simulink model "anti_condensation_control"  (R2025a)
settings: Solver=FixedStepDiscrete  StartTime=0.0  StopTime=5400  FixedStep=0.5  RelTol=1e-3
model workspace (MAT data in the model file):
  C_th = 700
  P_loss0 = 55
  R_th0 = 0.48
  T_mod0 = 27
  V_max = 880
  V_min = 580
  V_nom = 620
  dT_2nd = 8
  dT_th = 5
  dV_step = 15
  fan_nom = 100
undefined symbols (not defined in the file or in its folder): DiscIntNeverNeededParam
settings Model: Creator=jicai  LastModifiedBy=jicai

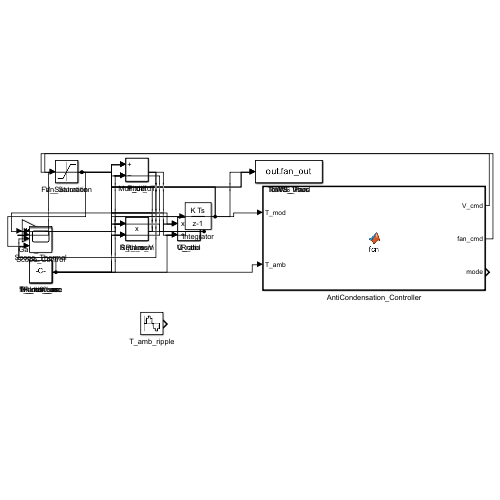
[thumbnail: Simulink's stored preview of the top-level diagram]
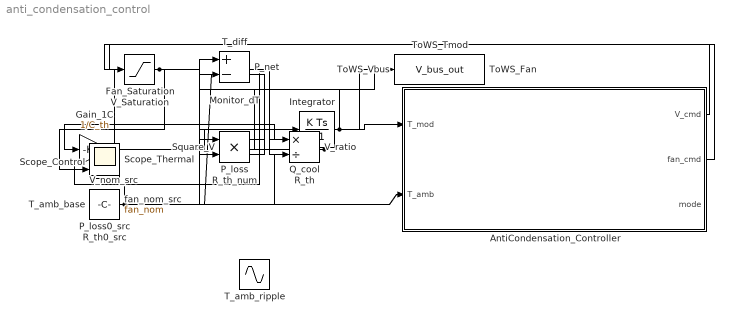
== system anti_condensation_control ==
  AntiCondensation_Controller : MATLAB Function  TreatAsAtomicUnit=on
  Fan_Saturation : Saturate  UpperLimit=100  LowerLimit=15
  Gain_1C : Gain  Gain=1/C_th
  Integrator : DiscreteIntegrator  InitialCondition=T_mod0  SampleTime=0.5  ICPrevOutput=DiscIntNeverNeededParam  ICPrevScaledInput=DiscIntNeverNeededParam
  Monitor_dT : Sum  Inputs=+-
  P_loss : Product  Inputs=**
  P_loss0_src : Constant  Value=P_loss0
  P_net : Sum  Inputs=+-
  Q_cool : Product  Inputs=*/
  R_th : Product  Inputs=*/
  R_th0_src : Constant  Value=R_th0
  R_th_num : Product  Inputs=**
  Scope_Control : Scope  NumInputPorts=2
  Scope_Thermal : Scope  NumInputPorts=3
  Square_V : Product  Inputs=**
  T_amb_base : Constant  Value=38
  T_amb_ripple : Sin  Amplitude=1.2  Frequency=0.00628  SampleTime=0.5
  T_diff : Sum  Inputs=+-
  ToWS_Fan : ToWorkspace  VariableName=fan_out  SaveFormat=Timeseries  SampleTime=-1
  ToWS_Tmod : ToWorkspace  VariableName=T_mod_out  SaveFormat=Timeseries  SampleTime=-1
  ToWS_Vbus : ToWorkspace  VariableName=V_bus_out  SaveFormat=Timeseries  SampleTime=-1
  V_Saturation : Saturate  UpperLimit=V_max  LowerLimit=V_min
  V_nom_src : Constant  Value=V_nom
  V_ratio : Product  Inputs=*/
  fan_nom_src : Constant  Value=fan_nom
  wires:
  T_amb_base/1 -> Monitor_dT/2, AntiCondensation_Controller/2(T_amb), T_diff/2, Scope_Thermal/2
  Integrator/1 -> AntiCondensation_Controller/1(T_mod), T_diff/1, Monitor_dT/1, Scope_Thermal/1, ToWS_Tmod/1
  AntiCondensation_Controller/1(V_cmd) -> V_Saturation/1
  AntiCondensation_Controller/2(fan_cmd) -> Fan_Saturation/1
  V_Saturation/1 -> V_ratio/1, Scope_Control/1, ToWS_Vbus/1
  V_nom_src/1 -> V_ratio/2
  V_ratio/1 -> Square_V/1, Square_V/2
  Square_V/1 -> P_loss/1
  P_loss0_src/1 -> P_loss/2
  R_th0_src/1 -> R_th_num/1
  fan_nom_src/1 -> R_th_num/2
  R_th_num/1 -> R_th/1
  Fan_Saturation/1 -> R_th/2, Scope_Control/2, ToWS_Fan/1
  T_diff/1 -> Q_cool/1
  R_th/1 -> Q_cool/2
  P_loss/1 -> P_net/1
  Q_cool/1 -> P_net/2
  P_net/1 -> Gain_1C/1
  Gain_1C/1 -> Integrator/1
  Monitor_dT/1 -> Scope_Thermal/3

== matlab function anti_condensation_control/AntiCondensation_Controller ==
  data: T_mod input; V_cmd output; T_amb input; fan_cmd output; mode output
function [V_cmd, fan_cmd, mode] = fcn(T_mod, T_amb)
persistent V_cur
persistent fan_cur
persistent tick
if isempty(V_cur)
    V_cur = 620;
    fan_cur = 100;
    tick = 0;
end
tick = tick + 1;
mode = int32(0);
if tick >= 40
    tick = 0;
    deltaT = T_amb - T_mod;
    if deltaT > 5
        if deltaT > 8
            V_cur = min(V_cur+15, 880);
            fan_cur = max(fan_cur-12, 15);
            mode = int32(2);
        else
            V_cur = min(V_cur+15, 880);
            mode = int32(1);
        end
    else
        if V_cur > 625
            V_cur = max(620, V_cur-9);
        end
        if fan_cur < 97
            fan_cur = min(100, fan_cur+6);
        end
        mode = int32(0);
    end
end
V_cmd = V_cur;
fan_cmd = fan_cur;
end
